simulink library "MEKF_lib"  (R2018b)
settings: Solver=VariableStepAuto  StartTime=0.0  StopTime=10.0  RelTol=1e-3
undefined symbols (not defined in the file or in its folder): fswParams
libraries: CrossProdMatrix_lib x4, sharedutil x2, aerolibutil x2, parallel_protection_lib x1, Triad_lib x1
settings Model: Creator=kylle  LastModifiedBy=Taylor

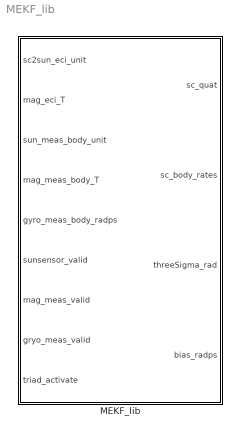
== system MEKF_lib ==
  MEKF_lib : Subsystem  TreatAsAtomicUnit=on
      settings: RTWFcnNameOpts=Use subsystem name  RTWFileNameOpts=Use subsystem name

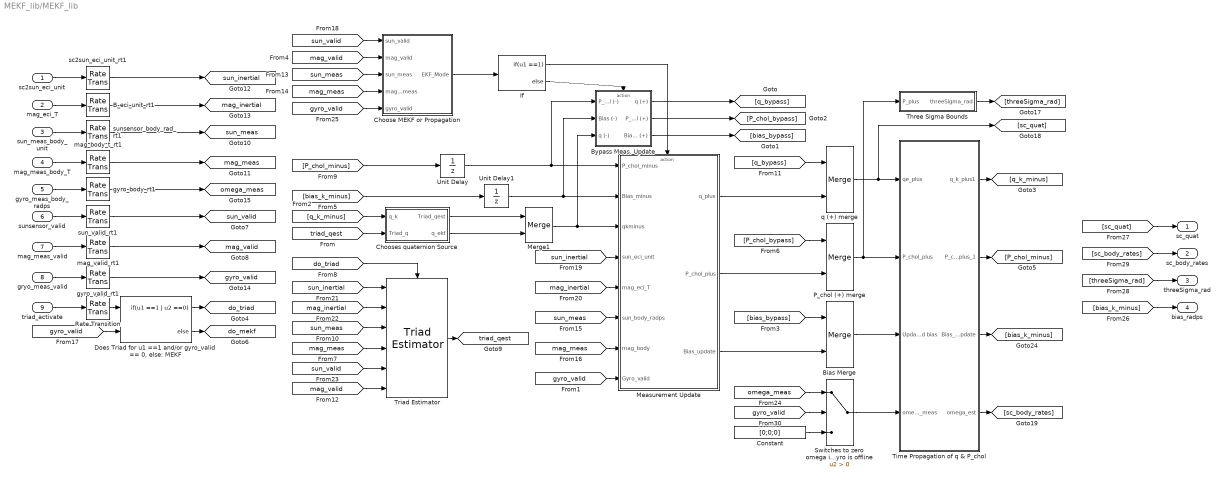
== system MEKF_lib/MEKF_lib ==
  sc2sun_eci_unit : Inport
  mag_eci_T : Inport  Port=2
  sun_meas_body_unit : Inport  Port=3
  mag_meas_body_T : Inport  Port=4
  gyro_meas_body_radps : Inport  Port=5
  sunsensor_valid : Inport  Port=6
  mag_meas_valid : Inport  Port=7
  gryo_meas_valid : Inport  Port=8
  triad_activate : Inport  Port=9
  B_eci_unit_rt1 : RateTransition  InitialCondition=fswParams.estimation.ic.B_eci_unit_rt  OutPortSampleTime=fswParams.sample_time_s
  Bias Merge : Merge
  Bypass Meas. Update : Subsystem  TreatAsAtomicUnit=on
  Choose MEKF or Propagation : Subsystem
  Chooses quaternion Source : Subsystem
  Constant : Constant  Value=[0;0;0]
  "Does Triad for u1 ==1 and/or gyro_valid == 0, else: MEKF" : If  NumInputs=2  IfExpression=u1 ==1 | u2 ==0
  If : If  IfExpression=u1 ==1
  Measurement Update : Subsystem  TreatAsAtomicUnit=on
  Merge1 : Merge
  P_chol (+) merge : Merge
  Rate Transition : RateTransition  InitialCondition=fswParams.estimation.ic.triad_input_rt  OutPortSampleTime=fswParams.sample_time_s
  "Switches to zero omega if Gyro is offline " : Switch  Criteria=u2 > Threshold
  Three Sigma Bounds : Subsystem
  Time Propagation of q & P_chol : Subsystem
  Triad Estimator : Triad_lib/Triad Estimator  SystemSampleTime=-1
  Unit Delay : UnitDelay  InitialCondition=fswParams.estimation.ic.Pchol_init  SampleTime=fswParams.sample_time_s
  Unit Delay1 : UnitDelay  InitialCondition=fswParams.estimation.ic.Beta_init  SampleTime=fswParams.sample_time_s
  gyro_body_rt1 : RateTransition  InitialCondition=fswParams.estimation.ic.gyro_meas_rt  OutPortSampleTime=fswParams.sample_time_s
  gyro_valid_rt1 : RateTransition  InitialCondition=fswParams.estimation.ic.gyro_valid_rt  OutPortSampleTime=fswParams.sample_time_s
  mag_body_t_rt1 : RateTransition  InitialCondition=fswParams.estimation.ic.mag_body_rt  OutPortSampleTime=fswParams.sample_time_s
  mag_valid_rt1 : RateTransition  InitialCondition=fswParams.estimation.ic.mag_valid_rt  OutPortSampleTime=fswParams.sample_time_s
  q (+) merge : Merge
  sc2sun_eci_unit_rt1 : RateTransition  InitialCondition=fswParams.estimation.ic.sc2sun_eci_unit_rt  OutPortSampleTime=fswParams.sample_time_s
  sun_valid_rt1 : RateTransition  InitialCondition=fswParams.estimation.ic.sun_valid_rt  OutPortSampleTime=fswParams.sample_time_s
  sunsensor_body_rad_rt1 : RateTransition  InitialCondition=fswParams.estimation.ic.sunsensor_body_rad_rt  OutPortSampleTime=fswParams.sample_time_s
  sc_quat : Outport
  sc_body_rates : Outport  Port=2
  "threeSigma_rad " : Outport  Port=3
  bias_radps : Outport  Port=4
  tag scope: do_mekf=global, do_triad=global, gyro_valid=global, mag_inertial=global, mag_meas=global, mag_valid=global, omega_meas=global, sun_inertial=global, sun_meas=global, sun_valid=global, triad_qest=global
  wires:
  Measurement Update/2(P_chol_plus) -> P_chol (+) merge/2
  Measurement Update/3(Bias_update) -> Bias Merge/2
  Measurement Update/1(q_plus) -> q (+) merge/2
  [gyro_valid] -> "Switches to zero omega if Gyro is offline "/2
  Choose MEKF or Propagation/1(EKF_Mode) -> If/1
  Bias Merge/1 -> Time Propagation of q & P_chol/3(Updated bias)
  "Switches to zero omega if Gyro is offline "/1 -> Time Propagation of q & P_chol/4(omega_meas)
  [sc_body_rates] -> sc_body_rates/1
  Time Propagation of q & P_chol/4(omega_est) -> [sc_body_rates]
  [threeSigma_rad] -> "threeSigma_rad "/1
  Three Sigma Bounds/1(threeSigma_rad) -> [threeSigma_rad]
  [sc_quat] -> sc_quat/1
  [bias_k_minus] -> bias_radps/1
  [gyro_valid] -> Choose MEKF or Propagation/5(gyro_valid)
  [gyro_valid] -> "Does Triad for u1 ==1 and/or gyro_valid == 0, else: MEKF"/2
  [mag_inertial] -> Triad Estimator/2
  [mag_valid] -> Triad Estimator/6
  [sun_inertial] -> Triad Estimator/1
  [mag_meas] -> Triad Estimator/4
  [sun_valid] -> Triad Estimator/5
  [do_triad] -> Triad Estimator/Action
  [sun_meas] -> Triad Estimator/3
  [mag_meas] -> Choose MEKF or Propagation/4(mag_meas)
  [sun_meas] -> Choose MEKF or Propagation/3(sun_meas)
  [mag_valid] -> Choose MEKF or Propagation/2(mag_valid)
  [sun_valid] -> Choose MEKF or Propagation/1(sun_valid)
  [gyro_valid] -> Measurement Update/8(Gyro_valid)
  [triad_qest] -> Chooses quaternion Source/2(Triad_q)
  Chooses quaternion Source/2(q_ekf) -> Merge1/2
  Chooses quaternion Source/1(Triad_qest) -> Merge1/1
  [q_k_minus] -> Chooses quaternion Source/1(q_k)
  Triad Estimator/1 -> [triad_qest]
  [sun_inertial] -> Measurement Update/4(sun_eci_unit)
  [mag_inertial] -> Measurement Update/5("mag_eci_T ")
  [omega_meas] -> "Switches to zero omega if Gyro is offline "/1
  gyro_body_rt1/1 -> [omega_meas]
  gyro_valid_rt1/1 -> [gyro_valid]
  B_eci_unit_rt1/1 -> [mag_inertial]
  sc2sun_eci_unit_rt1/1 -> [sun_inertial]
  Merge1/1 -> Measurement Update/3(qkminus), Bypass Meas. Update/3(q (-))
  Unit Delay1/1 -> Measurement Update/2(Bias_minus), Bypass Meas. Update/2(Bias (-))
  Unit Delay/1 -> Bypass Meas. Update/1(P_chol (-)), Measurement Update/1(P_chol_minus)
  mag_valid_rt1/1 -> [mag_valid]
  sun_valid_rt1/1 -> [sun_valid]
  [mag_meas] -> Measurement Update/7(mag_body)
  mag_body_t_rt1/1 -> [mag_meas]
  sunsensor_body_rad_rt1/1 -> [sun_meas]
  [sun_meas] -> Measurement Update/6(sun_body_radps)
  gyro_meas_body_radps/1 -> gyro_body_rt1/1
  mag_meas_valid/1 -> mag_valid_rt1/1
  sunsensor_valid/1 -> sun_valid_rt1/1
  "Does Triad for u1 ==1 and/or gyro_valid == 0, else: MEKF"/2 -> [do_mekf]
  "Does Triad for u1 ==1 and/or gyro_valid == 0, else: MEKF"/1 -> [do_triad]
  triad_activate/1 -> Rate Transition/1
  Rate Transition/1 -> "Does Triad for u1 ==1 and/or gyro_valid == 0, else: MEKF"/1
  sun_meas_body_unit/1 -> sunsensor_body_rad_rt1/1
  mag_meas_body_T/1 -> mag_body_t_rt1/1
  mag_eci_T/1 -> B_eci_unit_rt1/1
  sc2sun_eci_unit/1 -> sc2sun_eci_unit_rt1/1
  Time Propagation of q & P_chol/1(q_k_plus1) -> [q_k_minus]
  Time Propagation of q & P_chol/2(P_chol_plus_1) -> [P_chol_minus]
  If/1 -> Measurement Update/Action
  If/2 -> Bypass Meas. Update/Action
  [bias_k_minus] -> Unit Delay1/1
  [P_chol_minus] -> Unit Delay/1
  Bypass Meas. Update/1(q (+)) -> [q_bypass]
  [q_bypass] -> q (+) merge/1
  [bias_bypass] -> Bias Merge/1
  Bypass Meas. Update/2(P_chol (+)) -> [P_chol_bypass]
  Bypass Meas. Update/3(Bias (+)) -> [bias_bypass]
  gryo_meas_valid/1 -> gyro_valid_rt1/1
  Constant/1 -> "Switches to zero omega if Gyro is offline "/3
  P_chol (+) merge/1 -> Time Propagation of q & P_chol/2(P_chol_plus), Three Sigma Bounds/1(P_plus)
  [P_chol_bypass] -> P_chol (+) merge/1
  Time Propagation of q & P_chol/3(Bias_Update) -> [bias_k_minus]
  q (+) merge/1 -> Time Propagation of q & P_chol/1(qe_plus), [sc_quat]

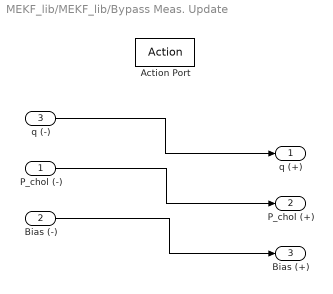
== system MEKF_lib/MEKF_lib/Bypass Meas. Update ==
  P_chol (-) : Inport
  Bias (-) : Inport  Port=2
  q (-) : Inport  Port=3
  Action Port : ActionPort
  q (+) : Outport
  P_chol (+) : Outport  Port=2
  Bias (+) : Outport  Port=3
  wires:
  P_chol (-)/1 -> P_chol (+)/1
  Bias (-)/1 -> Bias (+)/1
  q (-)/1 -> q (+)/1

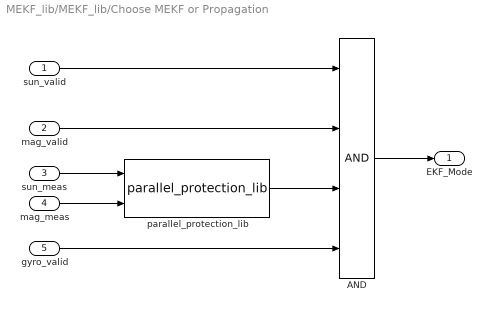
== system MEKF_lib/MEKF_lib/Choose MEKF or Propagation ==
  sun_valid : Inport
  mag_valid : Inport  Port=2
  sun_meas : Inport  Port=3
  mag_meas : Inport  Port=4
  gyro_valid : Inport  Port=5
  AND : Logic  Inputs=4  AllPortsSameDT=off  OutDataTypeStr=boolean
  parallel_protection_lib : parallel_protection_lib/parallel_protection_lib  min_angle_deg=1.5
  EKF_Mode : Outport
  wires:
  gyro_valid/1 -> AND/4
  mag_meas/1 -> parallel_protection_lib/2
  sun_meas/1 -> parallel_protection_lib/1
  mag_valid/1 -> AND/2
  sun_valid/1 -> AND/1
  AND/1 -> EKF_Mode/1
  parallel_protection_lib/1 -> AND/3

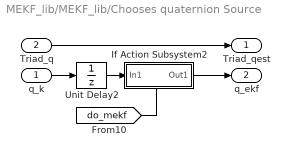
== system MEKF_lib/MEKF_lib/Chooses quaternion Source ==
  q_k : Inport
  Triad_q : Inport  Port=2
  If Action Subsystem2 : Subsystem  TreatAsAtomicUnit=on
  Unit Delay2 : UnitDelay  InitialCondition=fswParams.estimation.ic.quat_est_init  SampleTime=fswParams.sample_time_s
  Triad_qest : Outport
  q_ekf : Outport  Port=2
  wires:
  Triad_q/1 -> Triad_qest/1
  If Action Subsystem2/1(Out1) -> q_ekf/1
  q_k/1 -> Unit Delay2/1
  [do_mekf] -> If Action Subsystem2/Action
  Unit Delay2/1 -> If Action Subsystem2/1(In1)

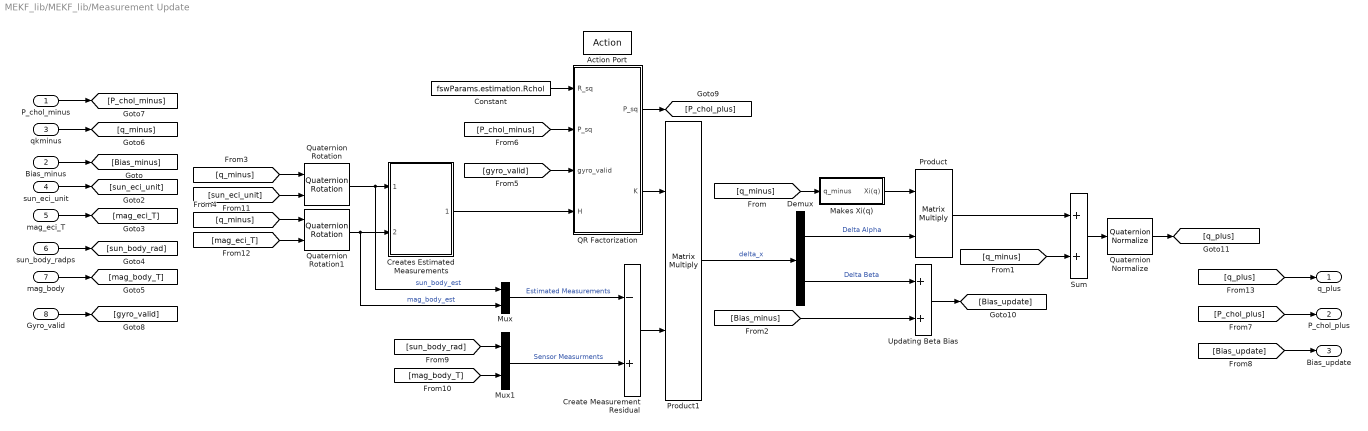
== system MEKF_lib/MEKF_lib/Measurement Update ==
  P_chol_minus : Inport
  Bias_minus : Inport  Port=2
  qkminus : Inport  Port=3
  sun_eci_unit : Inport  Port=4
  "mag_eci_T " : Inport  Port=5
  sun_body_radps : Inport  Port=6
  mag_body : Inport  Port=7
  Gyro_valid : Inport  Port=8
  Action Port : ActionPort
  Constant : Constant  Value=fswParams.estimation.Rchol  VectorParams1D=off
  Create Measurement Residual : Sum  Inputs=-+
  Creates Estimated Measurements : Subsystem
  Demux : Demux  Outputs=2
  Makes Xi(q) : Subsystem
  Mux : Mux  Inputs=2
  Mux1 : Mux  Inputs=2
  Product : Product  Inputs=**  Multiplication=Matrix(*)
  Product1 : Product  Multiplication=Matrix(*)
  QR Factorization : MATLAB Function  TreatAsAtomicUnit=on
  Quaternion Normalize : sharedutil/Quaternion Normalize  aMode=aMode
      settings: SourceProductName=Aerospace Blockset  SourceProductBaseCode=AE
  Quaternion Rotation : aerolibutil/Quaternion Rotation
  Quaternion Rotation1 : aerolibutil/Quaternion Rotation
  Sum : Sum
  "Updating Beta Bias " : Sum
  q_plus : Outport
  P_chol_plus : Outport  Port=2
  Bias_update : Outport  Port=3
  wires:
  [q_plus] -> q_plus/1
  Quaternion Normalize/1 -> [q_plus]
  [mag_eci_T] -> Quaternion Rotation1/2
  [sun_eci_unit] -> Quaternion Rotation/2
  [mag_body_T] -> Mux1/2
  [sun_body_rad] -> Mux1/1
  Gyro_valid/1 -> [gyro_valid]
  [Bias_update] -> Bias_update/1
  "Updating Beta Bias "/1 -> [Bias_update]
  [P_chol_plus] -> P_chol_plus/1
  QR Factorization/1(P_sq) -> [P_chol_plus]
  [P_chol_minus] -> QR Factorization/2("P_sq ")
  [gyro_valid] -> QR Factorization/3(gyro_valid)
  P_chol_minus/1 -> [P_chol_minus]
  mag_body/1 -> [mag_body_T]
  "mag_eci_T "/1 -> [mag_eci_T]
  sun_eci_unit/1 -> [sun_eci_unit]
  sun_body_radps/1 -> [sun_body_rad]
  [q_minus] -> Quaternion Rotation1/1
  [q_minus] -> Quaternion Rotation/1
  [Bias_minus] -> "Updating Beta Bias "/2
  Bias_minus/1 -> [Bias_minus]
  Constant/1 -> QR Factorization/1(R_sq)
  QR Factorization/2(K) -> Product1/1
  Creates Estimated Measurements/1(H_matrix) -> QR Factorization/4(H)
  [q_minus] -> Makes Xi(q)/1(q_minus)
  qkminus/1 -> [q_minus]
  Quaternion Rotation/1 -> Creates Estimated Measurements/1(sun_body_hat), Mux/1  "sun_body_est"
  Quaternion Rotation1/1 -> Creates Estimated Measurements/2(mag_body_hat), Mux/2  "mag_body_est"
  Create Measurement Residual/1 -> Product1/2
  Makes Xi(q)/1(Xi(q)) -> Product/1
  Demux/1 -> Product/2  "Delta Alpha"
  Product1/1 -> Demux/1  "delta_x"
  Product/1 -> Sum/1
  Sum/1 -> Quaternion Normalize/1
  Mux/1 -> Create Measurement Residual/1  "Estimated Measurements"
  Demux/2 -> "Updating Beta Bias "/1  "Delta Beta"
  Mux1/1 -> Create Measurement Residual/2  "Sensor Measurments"
  [q_minus] -> Sum/2

== system MEKF_lib/MEKF_lib/Three Sigma Bounds ==
  P_plus : Inport
  Abs : Abs
  Extract Diagonal : S-Function  FunctionName=sdspdiag2  Parameters=mode  SFunctionDeploymentMode=off  EnableBusSupport=off  mask(Extract Diagonal){}
      mask help: Extract the main diagonal of a full matrix.
      mask init:
      | mode = 2;
      | x = [.58 .87 NaN 0.12 0.45 0.45 0.12 0.12 NaN 0.525 0.525 0.475 0.475 0.525 0.525 0.565 0.525 ];
      | y = [ 0.8 0.2 NaN 0.2 0.2 0.8 0.8 0.2 NaN 0.435 0.475 0.475 0.525 0.525 0.565 0.5 0.435 ];
      mask Help: eval('blocksethelp');
      mask Display:
      | plot(x,y);
      | port_label('input',1,'A');
      | port_label('output',1,'D');
  multiply : Gain  Gain=3
  threeSigma_rad : Outport
  wires:
  Extract Diagonal/1 -> Abs/1
  Abs/1 -> multiply/1  "sigma"
  P_plus/1 -> Extract Diagonal/1
  multiply/1 -> threeSigma_rad/1

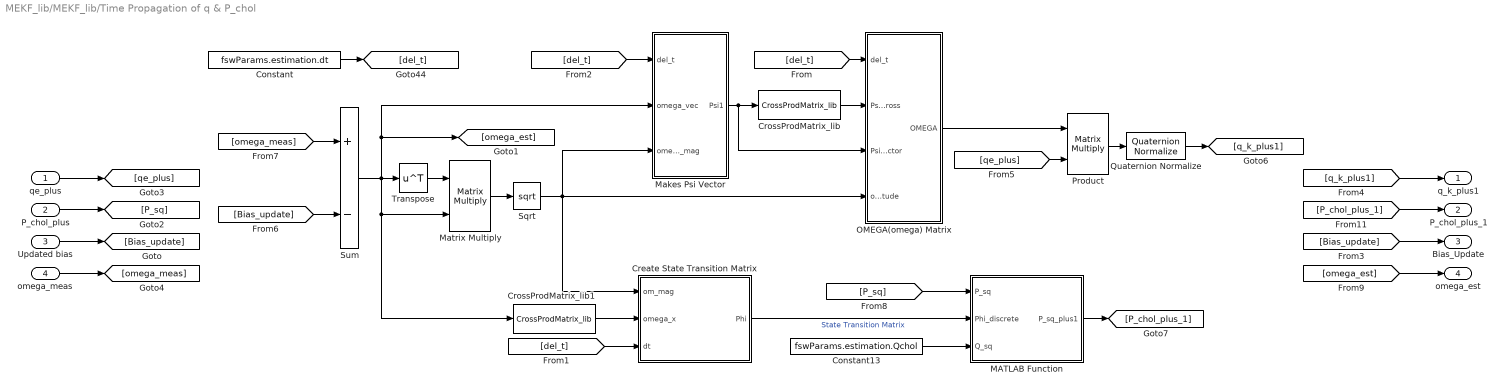
== system MEKF_lib/MEKF_lib/Time Propagation of q & P_chol ==
  qe_plus : Inport
  P_chol_plus : Inport  Port=2
  Updated bias : Inport  Port=3
  omega_meas : Inport  Port=4
  Constant : Constant  Value=fswParams.estimation.dt
  Constant13 : Constant  Value=fswParams.estimation.Qchol  VectorParams1D=off
  Create State Transition Matrix : MATLAB Function  TreatAsAtomicUnit=on
  CrossProdMatrix_lib : CrossProdMatrix_lib/CrossProdMatrix_lib  SystemSampleTime=-1
  CrossProdMatrix_lib1 : CrossProdMatrix_lib/CrossProdMatrix_lib  SystemSampleTime=-1
  MATLAB Function : MATLAB Function  TreatAsAtomicUnit=on
  Makes Psi Vector : Subsystem
  Matrix Multiply : Product  Multiplication=Matrix(*)
  OMEGA(omega) Matrix : Subsystem
  Product : Product  Multiplication=Matrix(*)
  Quaternion Normalize : sharedutil/Quaternion Normalize  aMode=aMode
      settings: SourceProductName=Aerospace Blockset  SourceProductBaseCode=AE
  Sqrt : Sqrt  SaturateOnIntegerOverflow=on
  Sum : Sum  Inputs=+-
  Transpose : Math  Operator=transpose  SaturateOnIntegerOverflow=on
  q_k_plus1 : Outport
  P_chol_plus_1 : Outport  Port=2
  Bias_Update : Outport  Port=3
  omega_est : Outport  Port=4
  wires:
  Create State Transition Matrix/1(Phi) -> MATLAB Function/2(Phi_discrete)  "State Transition Matrix"
  Constant13/1 -> MATLAB Function/3(Q_sq)
  [P_sq] -> MATLAB Function/1(P_sq)
  [P_chol_plus_1] -> P_chol_plus_1/1
  MATLAB Function/1(P_sq_plus1) -> [P_chol_plus_1]
  [q_k_plus1] -> q_k_plus1/1
  Quaternion Normalize/1 -> [q_k_plus1]
  [omega_meas] -> Sum/1
  [Bias_update] -> Sum/2
  omega_meas/1 -> [omega_meas]
  P_chol_plus/1 -> [P_sq]
  Updated bias/1 -> [Bias_update]
  [qe_plus] -> Product/2
  qe_plus/1 -> [qe_plus]
  [omega_est] -> omega_est/1
  [Bias_update] -> Bias_Update/1
  OMEGA(omega) Matrix/1(OMEGA) -> Product/1
  CrossProdMatrix_lib/1 -> OMEGA(omega) Matrix/2(Psi_cross)
  Makes Psi Vector/1(Psi1) -> OMEGA(omega) Matrix/3(Psi_vector), CrossProdMatrix_lib/1
  [del_t] -> OMEGA(omega) Matrix/1(del_t)
  CrossProdMatrix_lib1/1 -> Create State Transition Matrix/2(omega_x)
  Sqrt/1 -> Create State Transition Matrix/1(om_mag), Makes Psi Vector/3(omega_mag), OMEGA(omega) Matrix/4(omega_magnitude)
  Transpose/1 -> Matrix Multiply/1
  Matrix Multiply/1 -> Sqrt/1
  Constant/1 -> [del_t]
  Sum/1 -> Makes Psi Vector/2(omega_vec), [omega_est], CrossProdMatrix_lib1/1, Matrix Multiply/2, Transpose/1
  [del_t] -> Makes Psi Vector/1(del_t)
  [del_t] -> Create State Transition Matrix/3(dt)
  Product/1 -> Quaternion Normalize/1

== system MEKF_lib/MEKF_lib/Chooses quaternion Source/If Action Subsystem2 ==
  In1 : Inport
  Action Port : ActionPort
  Out1 : Outport
  wires:
  In1/1 -> Out1/1

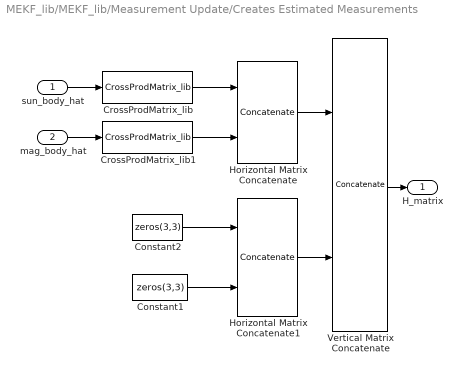
== system MEKF_lib/MEKF_lib/Measurement Update/Creates Estimated Measurements ==
  sun_body_hat : Inport
  mag_body_hat : Inport  Port=2
  Constant1 : Constant  Value=zeros(3,3)  VectorParams1D=off
  Constant2 : Constant  Value=zeros(3,3)  VectorParams1D=off
  CrossProdMatrix_lib : CrossProdMatrix_lib/CrossProdMatrix_lib  SystemSampleTime=-1
  CrossProdMatrix_lib1 : CrossProdMatrix_lib/CrossProdMatrix_lib  SystemSampleTime=-1
  Horizontal Matrix Concatenate : Concatenate  Mode=Multidimensional array
  Horizontal Matrix Concatenate1 : Concatenate  Mode=Multidimensional array
  Vertical Matrix Concatenate : Concatenate  Mode=Multidimensional array  ConcatenateDimension=2
  H_matrix : Outport
  wires:
  Constant1/1 -> Horizontal Matrix Concatenate1/2
  Constant2/1 -> Horizontal Matrix Concatenate1/1
  CrossProdMatrix_lib1/1 -> Horizontal Matrix Concatenate/2
  Horizontal Matrix Concatenate/1 -> Vertical Matrix Concatenate/1
  Horizontal Matrix Concatenate1/1 -> Vertical Matrix Concatenate/2
  sun_body_hat/1 -> CrossProdMatrix_lib/1
  CrossProdMatrix_lib/1 -> Horizontal Matrix Concatenate/1
  mag_body_hat/1 -> CrossProdMatrix_lib1/1
  Vertical Matrix Concatenate/1 -> H_matrix/1

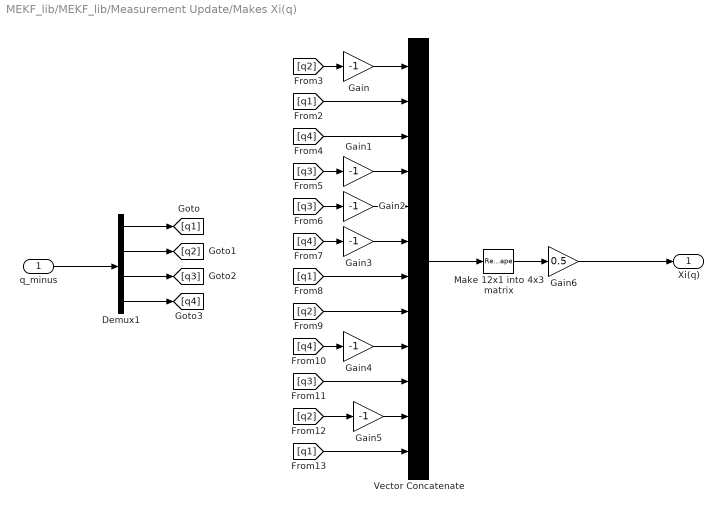
== system MEKF_lib/MEKF_lib/Measurement Update/Makes Xi(q) ==
  q_minus : Inport
  Demux1 : Demux
  Gain{,1..5} (6 alike) : Gain  Gain=-1
  Gain6 : Gain  Gain=0.5
  Make 12x1 into 4x3 matrix : Reshape  OutputDimensionality=Customize  OutputDimensions=[4,3]
  Vector Concatenate : Concatenate  NumInputs=12
  Xi(q) : Outport
  wires:
  Vector Concatenate/1 -> Make 12x1 into 4x3 matrix/1
  [q3] -> Gain2/1
  Gain3/1 -> Vector Concatenate/6
  [q1] -> Vector Concatenate/2
  Make 12x1 into 4x3 matrix/1 -> Gain6/1
  [q3] -> Gain1/1
  [q4] -> Gain3/1
  [q2] -> Gain/1
  [q3] -> Vector Concatenate/10
  Gain2/1 -> Vector Concatenate/5
  Gain1/1 -> Vector Concatenate/4
  Demux1/2 -> [q2]
  [q2] -> Vector Concatenate/8
  Demux1/1 -> [q1]
  Gain4/1 -> Vector Concatenate/9
  Demux1/3 -> [q3]
  [q4] -> Vector Concatenate/3
  [q1] -> Vector Concatenate/12
  Gain/1 -> Vector Concatenate/1
  [q2] -> Gain5/1
  [q4] -> Gain4/1
  Gain5/1 -> Vector Concatenate/11
  [q1] -> Vector Concatenate/7
  Demux1/4 -> [q4]
  q_minus/1 -> Demux1/1
  Gain6/1 -> Xi(q)/1

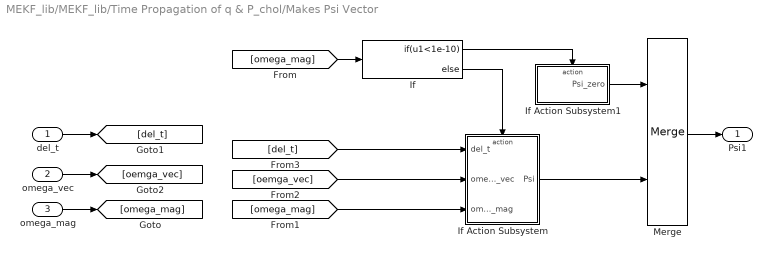
== system MEKF_lib/MEKF_lib/Time Propagation of q & P_chol/Makes Psi Vector ==
  del_t : Inport
  omega_vec : Inport  Port=2
  omega_mag : Inport  Port=3
  If : If  IfExpression=u1<1e-10
  If Action Subsystem : Subsystem  TreatAsAtomicUnit=on
  If Action Subsystem1 : Subsystem  TreatAsAtomicUnit=on
  Merge : Merge
  Psi1 : Outport
  wires:
  [del_t] -> If Action Subsystem/1(del_t)
  [oemga_vec] -> If Action Subsystem/2(omega_vec)
  del_t/1 -> [del_t]
  omega_vec/1 -> [oemga_vec]
  [omega_mag] -> If/1
  [omega_mag] -> If Action Subsystem/3(omega_mag)
  omega_mag/1 -> [omega_mag]
  Merge/1 -> Psi1/1
  If Action Subsystem1/1(Psi_zero) -> Merge/1
  If/1 -> If Action Subsystem1/Action
  If Action Subsystem/1(Psi) -> Merge/2
  If/2 -> If Action Subsystem/Action

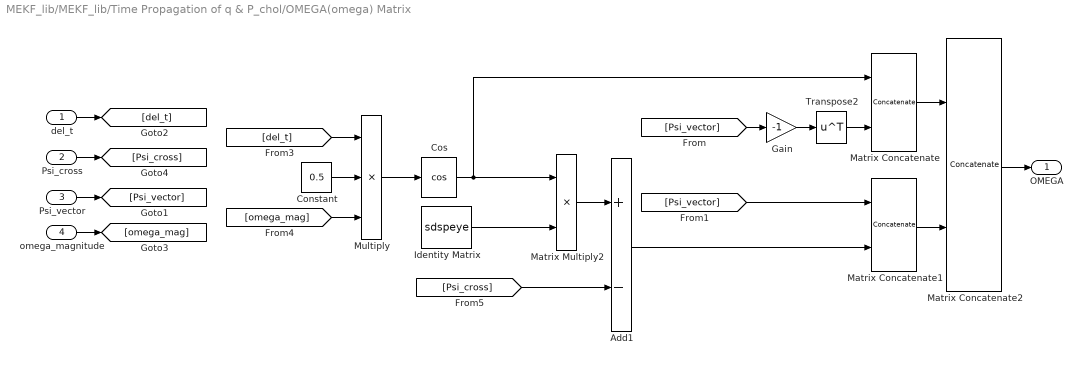
== system MEKF_lib/MEKF_lib/Time Propagation of q & P_chol/OMEGA(omega) Matrix ==
  del_t : Inport
  Psi_cross : Inport  Port=2
  Psi_vector : Inport  Port=3
  omega_magnitude : Inport  Port=4
  Add1 : Sum  Inputs=+-
  Constant : Constant  Value=0.5
  Cos : Trigonometry  Operator=cos
  Gain : Gain  Gain=-1
  Identity Matrix : S-Function  FunctionName=sdspeye  Parameters=Inherit,N,Ts,isCustomFloat,fxpIsSigned,dTypeID,fxpWordLength,fxpFracLength,1  SFunctionDeploymentMode=off  EnableBusSupport=off  mask(Identity Matrix){Inherit=off, N=3, Ts=fswParams.sample_time_s, additionalParams=off, allowOverrides=on, dataType=double, isSigned=on, wordLen=16, udDataType=sfix(16), fracBitsMode=Best precision, numFracBits=15, OutDataTypeStr=double, LastOutDataTypeStr=double}
      mask prompts: Inherit "Inherit output port attributes from input port"; N "Matrix size:"; Ts "Sample time:"; additionalParams "------- Show additional parameters --------"; allowOverrides "Allow overrides by DSP Fixed-Point Attributes blocks"; dataType "Output data type:"; isSigned "Signed"; wordLen "Word length:"; udDataType "User-defined data type (e.g. sfix(16), float('single')):"; fracBitsMode "Set fraction length in output to:"; numFracBits "Fraction length:"; OutDataTypeStr "Output data type:"; LastOutDataTypeStr "Last output data type:"
      mask help: Output an identity matrix. If the matrix size entered is a scalar, then the output will be a square (symmetric) identity matrix with the number of rows and columns both equal to the specified value. If the matrix size entered is a two-element vector [M N], then the output will be an asymmetric matrix with the number of rows equal to M, the number of columns equal to N, ones down the diagonal, and zeros elsewhere. This matches the syntax of the MATLAB function eye(N) and eye(M,N), respectively.
      mask init:
      | isCustomFloat =  0; % nice default
      | fxpIsSigned   =  1; % nice default
      | fxpWordLength =  8; % nice default
      | fxpFracLength =  0; % nice default
      | if Inherit
      |     dTypeID   = -3; % SAME_AS_INPUT
      | else
      |     dtRows            = dspblkGetDiscreteImpulseDTRowInfo();
      |     [dtInfo, dTypeID] = dspblkUDTMapperOutDType(gcbh, dtRows{1}, 'dataType', 1.0);
      |     isCustomFloat     = dtInfo.DataTypeIsCustomFloat;
      |     if ~isCustomFloat
      |         fxpIsSigned   = dtInfo.DataTypeIsSigned;
      |         fxpWordLength = dtInfo.DataTypeWordLength;
      |         fxpFracLength = dtInfo.DataTypeFracOrMantBits;
      |     end
      | end
      mask Help: eval('blocksethelp');
      mask Callback Inherit: dspblkeye
      mask TypeOptions dataType: double | single | int8 | uint8 | int16 | uint16 | int32 | uint32 | boolean | Fixed-point | User-defined | Inherit via back propagation
      mask TypeOptions fracBitsMode: Best precision | User-defined
      mask Display:
      | if Inherit
      |     disp('eye( )');
      | else
      |     disp(['eye(' , num2str(get_param(gcbh, 'N')), ')']);
      | end
  Matrix Concatenate : Concatenate  Mode=Multidimensional array  ConcatenateDimension=2
  Matrix Concatenate1 : Concatenate  Mode=Multidimensional array  ConcatenateDimension=2
  Matrix Concatenate2 : Concatenate  Mode=Multidimensional array
  Matrix Multiply2 : Product
  Multiply : Product  Inputs=3
  Transpose2 : Math  Operator=transpose  SaturateOnIntegerOverflow=on
  OMEGA : Outport
  wires:
  Identity Matrix/1 -> Matrix Multiply2/2
  [Psi_cross] -> Add1/2
  Psi_cross/1 -> [Psi_cross]
  [omega_mag] -> Multiply/3
  omega_magnitude/1 -> [omega_mag]
  [del_t] -> Multiply/1
  del_t/1 -> [del_t]
  [Psi_vector] -> Matrix Concatenate1/1
  [Psi_vector] -> Gain/1
  Psi_vector/1 -> [Psi_vector]
  Gain/1 -> Transpose2/1
  Constant/1 -> Multiply/2
  Transpose2/1 -> Matrix Concatenate/2
  Cos/1 -> Matrix Concatenate/1, Matrix Multiply2/1
  Matrix Concatenate/1 -> Matrix Concatenate2/1
  Matrix Concatenate1/1 -> Matrix Concatenate2/2
  Add1/1 -> Matrix Concatenate1/2
  Matrix Multiply2/1 -> Add1/1
  Multiply/1 -> Cos/1
  Matrix Concatenate2/1 -> OMEGA/1

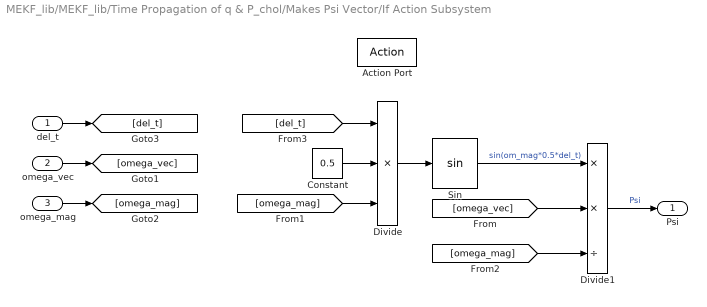
== system MEKF_lib/MEKF_lib/Time Propagation of q & P_chol/Makes Psi Vector/If Action Subsystem ==
  del_t : Inport
  omega_vec : Inport  Port=2
  omega_mag : Inport  Port=3
  Action Port : ActionPort
  Constant : Constant  Value=0.5
  Divide : Product  Inputs=***
  Divide1 : Product  Inputs=**/
  Sin : Trigonometry
  Psi : Outport
  wires:
  [del_t] -> Divide/1
  del_t/1 -> [del_t]
  [omega_mag] -> Divide1/3
  [omega_mag] -> Divide/3
  omega_mag/1 -> [omega_mag]
  [omega_vec] -> Divide1/2
  omega_vec/1 -> [omega_vec]
  Sin/1 -> Divide1/1  "sin(om_mag*0.5*del_t)"
  Divide/1 -> Sin/1
  Constant/1 -> Divide/2
  Divide1/1 -> Psi/1  "Psi"

== system MEKF_lib/MEKF_lib/Time Propagation of q & P_chol/Makes Psi Vector/If Action Subsystem1 ==
  Action Port : ActionPort
  Constant : Constant  Value=0
  Constant1 : Constant  Value=0
  Constant2 : Constant  Value=0
  Mux : Mux  Inputs=3
  Psi_zero : Outport
  wires:
  Mux/1 -> Psi_zero/1
  Constant2/1 -> Mux/3
  Constant1/1 -> Mux/2
  Constant/1 -> Mux/1

== matlab function MEKF_lib/Time Propagation of q & P_chol/MATLAB Function ==
  data: P_sq input; Phi_discrete input; Q_sq input; P_sq_plus1 output
function P_sq_plus1  = time_qr(P_sq,Phi_discrete,Q_sq)
%#codegen

C = [P_sq'*Phi_discrete';Q_sq'];
          [~,R2] = qr(C);
         P_sq_plus1 = R2(1:6,1:6)';

end

== matlab function MEKF_lib/Measurement Update/QR Factorization ==
  data: P_sq output; R_sq input; K output; P_sq input; gyro_valid input; H input
function [P_sq,K] = A_QR(R_sq,P_sq, gyro_valid,H)
%#codegen
[nr,~] = size(R_sq);
[np,~] = size(P_sq);
A_QR = [R_sq',zeros(nr,np);(P_sq')*H', P_sq'];

[~,R] = qr(A_QR);
        P_sq = R(7:12,7:12)'; %Updated P_sq
        K_bar = R(1:6,7:12)';    
        Innovation_sq = R(1:6,1:6)';
        
        K = K_bar/(Innovation_sq);
        
        if( gyro_valid == 0 )
    K(4:6,:) = zeros(3,6); %this is done so that we do not update bias based
                            % on false gyro readings
        end
end

== matlab function MEKF_lib/Time Propagation of q & P_chol/Create State Transition Matrix ==
  data: om_mag input; omega_x input; dt input; Phi output
function Phi = Phi_disc(om_mag,omega_x,dt)
%#codegen
% State Transition Matrix
w_n     = om_mag;
w_skew  = omega_x;

if( w_n < 1e-10 )
    Phi = [ eye(3)     -eye(3)*dt;
            zeros(3,3)  eye(3) ];
else
    Phi_11  = eye(3) - w_skew*(sin(w_n*dt)/w_n) + ...
                                        w_skew^2*(1 - cos(w_n*dt))/w_n^2;
    Phi_12  = w_skew*(1 - cos(w_n*dt))/w_n^2 - eye(3)*dt - ...
                                    w_skew^2*(w_n*dt - sin(w_n*dt))/w_n^3;
    Phi_21  = zeros(3,3);    
    Phi_22  = eye(3);    
    Phi     = [ Phi_11 Phi_12;
                Phi_21 Phi_22 ];
end
